simulink model "controlMCUSlugsMKII"  (Simulink 6.6)
settings: Solver=FixedStepDiscrete  StartTime=0.0  StopTime=10.0  FixedStep=0.01  RelTol=1e-3
InitFcn:
  | mcuInit
values from neighbouring files (symbols this model uses):
  apSampleTime = 0.01    [mcuInit.m]
  derivativesConstant = 5    [mcuInit.m]
  T = 0.01    [mcuInit.m]
undefined symbols (not defined in the file or in its folder): bankCommandLimit, baseHeight, bda, bde, bdr, bdt, bICda, bICde, bICdr, bICdt, controlMCUInit, daLimit, deLimit, drLimit, dtLimit, getAccBias, getAccels, getAttitude, getMidLevelCommands, getPassValues, getPidIdx, getVned, getWP, getXYZ, gsRead, ISA_g, lowRateTelemetryMavlink, mda, mde, mdr, mdt, mICda, mICde, mICdr, mICdt, pitchCommandLimit, protDecodeMavlink, readIpc, send2GS, setCurrentCommands, setDiagnosticFloat, setDiagnosticShort, setLogFloat1, setLogFloat2, setNavLat, setNavLong, setNavNav, u1, u2, updateEuler, updateLoad, updatePQR, updatePWM, updatePWM2, y1
libraries: dsPICdrivers x85, simulink x79, SLUGS_Library x23, aerolibconvert2 x5, aerolibutil x3
(part 3 of 5)

== system controlMCUSlugsMKII/Inner Loop/ Navigation/Longitudinal Channel/Protect NaNs ==
  In1 : Inport
  Integer Delay3 : simulink/Discrete/Integer Delay  Orientation=left  vinit=0.0  samptime=T  NumDelays=1
  Relational Operator2 : RelationalOperator  Operator===  LogicOutDataTypeMode=Specify via dialog
  Switch3 : Switch  Criteria=u2 > Threshold  Threshold=0.3  SampleTime=.01
  Out1 : Outport  Orientation=down
  wires:
  Relational Operator2/1 -> Switch3/2
  In1/1 -> Switch3/1, Relational Operator2/1, Relational Operator2/2
  Switch3/1 -> Integer Delay3/1, Out1/1
  Integer Delay3/1 -> Switch3/3

== system controlMCUSlugsMKII/Inner Loop/ Navigation/Longitudinal Channel/Protect NaNs1 ==
  In1 : Inport
  Integer Delay3 : simulink/Discrete/Integer Delay  Orientation=left  vinit=0.0  samptime=T  NumDelays=1
  Relational Operator2 : RelationalOperator  Operator===  LogicOutDataTypeMode=Specify via dialog
  Switch3 : Switch  Criteria=u2 > Threshold  Threshold=0.3  SampleTime=.01
  Out1 : Outport  Orientation=down
  wires:
  Relational Operator2/1 -> Switch3/2
  In1/1 -> Switch3/1, Relational Operator2/1, Relational Operator2/2
  Switch3/1 -> Integer Delay3/1, Out1/1
  Integer Delay3/1 -> Switch3/3

== system controlMCUSlugsMKII/Inner Loop/ Navigation/Longitudinal Channel/Protect NaNs2 ==
  In1 : Inport
  Integer Delay3 : simulink/Discrete/Integer Delay  Orientation=left  vinit=0.0  samptime=T  NumDelays=1
  Relational Operator2 : RelationalOperator  Operator===  LogicOutDataTypeMode=Specify via dialog
  Switch3 : Switch  Criteria=u2 > Threshold  Threshold=0.3  SampleTime=.01
  Out1 : Outport  Orientation=down
  wires:
  Integer Delay3/1 -> Switch3/3
  Switch3/1 -> Out1/1, Integer Delay3/1
  In1/1 -> Relational Operator2/2, Relational Operator2/1, Switch3/1
  Relational Operator2/1 -> Switch3/2

== system controlMCUSlugsMKII/Inner Loop/ Navigation/Longitudinal Channel/Protect NaNs3 ==
  In1 : Inport
  Integer Delay3 : simulink/Discrete/Integer Delay  Orientation=left  vinit=0.0  samptime=T  NumDelays=1
  Relational Operator2 : RelationalOperator  Operator===  LogicOutDataTypeMode=Specify via dialog
  Switch3 : Switch  Criteria=u2 > Threshold  Threshold=0.3  SampleTime=.01
  Out1 : Outport  Orientation=down
  wires:
  Integer Delay3/1 -> Switch3/3
  Switch3/1 -> Out1/1, Integer Delay3/1
  In1/1 -> Relational Operator2/2, Relational Operator2/1, Switch3/1
  Relational Operator2/1 -> Switch3/2

== system controlMCUSlugsMKII/Inner Loop/ Navigation/Longitudinal Channel/Protect NaNs4 ==
  In1 : Inport
  Integer Delay3 : simulink/Discrete/Integer Delay  Orientation=left  vinit=0.0  samptime=T  NumDelays=1
  Relational Operator2 : RelationalOperator  Operator===  LogicOutDataTypeMode=Specify via dialog
  Switch3 : Switch  Criteria=u2 > Threshold  Threshold=0.3  SampleTime=.01
  Out1 : Outport  Orientation=down
  wires:
  Integer Delay3/1 -> Switch3/3
  Switch3/1 -> Out1/1, Integer Delay3/1
  In1/1 -> Relational Operator2/2, Relational Operator2/1, Switch3/1
  Relational Operator2/1 -> Switch3/2

== system controlMCUSlugsMKII/Inner Loop/ Navigation/Longitudinal Channel/Subsystem5 ==
  u : Inport
  C Function Call1 : dsPICdrivers/OTHERS/C Function Call  Tag=dsPIC_dsPIC_CFunctionCall  fctName='myCos'  INPUT_SIZE=1  INPUT1=real32  INPUT2=--  INPUT3=--  OUTPUT_SIZE=1  OUTPUT1=real32  SampleTime=-1  InputType=[ 7 ]  OutputType=[ 7 ]  FctDeclaration=extern real32_T myCos(real32_T u1);  FctCall=%y1 = myCos(%u1);  OrderingInOutPopup=None
  cos(u) : Outport
  wires:
  u/1 -> C Function Call1/1
  C Function Call1/1 -> cos(u)/1

== system controlMCUSlugsMKII/Inner Loop/ Navigation/Navigation/Compute Lateral Error ==
  N : Inport
  WP1 : Inport  Port=2
  UAV pos : Inport  Port=3
  Add : Sum  Inputs=+-  OutScaling=2^-10
  Subsystem3 : Subsystem  AncestorBlock=SLUGS_Library/Subsystem3
  Pe_lat : Outport
  wires:
  Subsystem3/1(x dot y) -> Pe_lat/1
  Add/1 -> Subsystem3/2(y)
  N/1 -> Subsystem3/1(x)
  UAV pos/1 -> Add/2
  WP1/1 -> Add/1

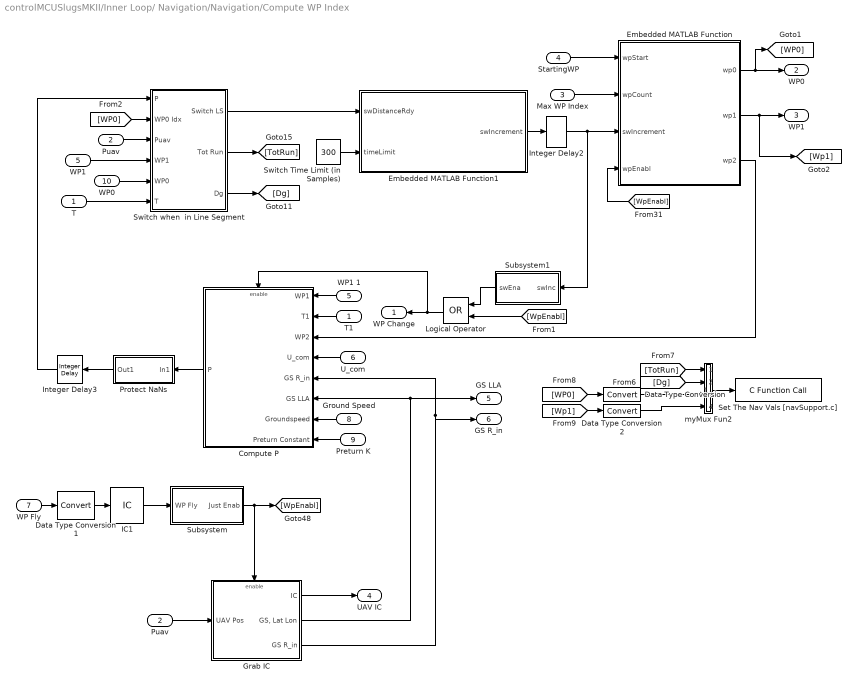
== system controlMCUSlugsMKII/Inner Loop/ Navigation/Navigation/Compute WP Index ==
  T1 : Inport  Orientation=left
  Puav : Inport  Port=2
  Max WP Index : Inport  Port=3
  StartingWP : Inport  Port=4
  "WP1 " : Inport  Port=5
  U_com : Inport  Orientation=left  Port=6
  WP Fly : Inport  Port=7
  Ground Speed : Inport  Orientation=left  Port=8
  Preturn K : Inport  Orientation=left  Port=9
  "WP0 " : Inport  Port=10
  Compute P : Subsystem  Orientation=left
  Data Type Conversion : DataTypeConversion  OutDataTypeMode=single
  Data Type Conversion1 : DataTypeConversion  OutDataTypeMode=double  SampleTime=apSampleTime
  Data Type Conversion2 : DataTypeConversion  OutDataTypeMode=single
  Embedded MATLAB Function : Stateflow chart
  Embedded MATLAB Function1 : Stateflow chart
  Grab IC : Subsystem  TreatAsAtomicUnit=on
  IC1 : InitialCondition  Value=0
  Integer Delay2 : simulink/Discrete/Integer Delay  vinit=1  samptime=-1  NumDelays=1
  Integer Delay3 : simulink/Discrete/Integer Delay  Orientation=left  vinit=50  samptime=-1  NumDelays=1
  Logical Operator : Logic  Orientation=left  Operator=OR  AllPortsSameDT=off  OutDataTypeMode=Boolean
  Protect NaNs : Subsystem  Orientation=left
  "Puav " : InportShadow  Port=2  LatchByCopyingInsideSignal=off
  Set The Nav Vals [navSupport.c] : dsPICdrivers/OTHERS/C Function Call  Tag=dsPIC_dsPIC_CFunctionCall  fctName='setNavNav'  INPUT_SIZE=4  INPUT1=real32  INPUT2=--  INPUT3=--  OUTPUT_SIZE=1  OUTPUT1=--  SampleTime=.01  InputType=[ 7 ]  OutputType=[ ]  FctDeclaration=extern void setNavNav(real32_T* u1);  FctCall=setNavNav(*%u1);  OrderingInOutPopup=None
  Subsystem : Subsystem
  Subsystem1 : Subsystem  Orientation=left
  Switch Time Limit (in Samples) : Constant  Value=300  OutDataTypeMode=single
  Switch when  in Line Segment : Subsystem
  "T " : InportShadow  Port=1  LatchByCopyingInsideSignal=off
  WP1 1 : InportShadow  Orientation=left  Port=5  LatchByCopyingInsideSignal=off
  myMux Fun2 : Stateflow chart
  WP Change : Outport  Orientation=left
  WP0 : Outport  Port=2
  WP1 : Outport  Port=3
  UAV IC : Outport  Port=4
  GS LLA : Outport  Port=5
  GS R_in : Outport  Port=6
  wires:
  Subsystem1/1(swEna) -> Logical Operator/1
  Switch Time Limit (in Samples)/1 -> Embedded MATLAB Function1/2(timeLimit)
  Switch when  in Line Segment/1(Switch LS) -> Embedded MATLAB Function1/1(swDistanceRdy)
  [WpEnabl] -> Logical Operator/2
  Embedded MATLAB Function1/1(swIncrement) -> Integer Delay2/1
  Grab IC/3(GS R_in) -> GS R_in/1, Compute P/5(GS R_in)
  Grab IC/2("GS, Lat Lon") -> GS LLA/1, Compute P/6(GS LLA)
  Logical Operator/1 -> WP Change/1, Compute P/Enable
  [WpEnabl] -> Embedded MATLAB Function/4(wpEnabl)
  IC1/1 -> Subsystem/1(WP Fly)
  Grab IC/1(IC) -> UAV IC/1
  "Puav "/1 -> Grab IC/1(UAV Pos)
  Subsystem/1(Just Enab) -> Grab IC/Enable, [WpEnabl]
  WP Fly/1 -> Data Type Conversion1/1
  U_com/1 -> Compute P/4(U_com)
  Compute P/1(P) -> Protect NaNs/1(In1)
  T1/1 -> Compute P/2(T1)
  WP1 1/1 -> Compute P/1(WP1)
  Embedded MATLAB Function/3(wp2) -> Compute P/3(WP2)
  Max WP Index/1 -> Embedded MATLAB Function/2(wpCount)
  StartingWP/1 -> Embedded MATLAB Function/1(wpStart)
  Embedded MATLAB Function/1(wp0) -> [WP0], WP0/1
  Embedded MATLAB Function/2(wp1) -> WP1/1, [Wp1]
  Data Type Conversion1/1 -> IC1/1
  Ground Speed/1 -> Compute P/7(Groundspeed)
  Preturn K/1 -> Compute P/8(Preturn Constant)
  [WP0] -> Switch when  in Line Segment/2(WP0 Idx)
  Puav/1 -> Switch when  in Line Segment/3(Puav)
  Integer Delay3/1 -> Switch when  in Line Segment/1(P)
  "WP1 "/1 -> Switch when  in Line Segment/4("WP1 ")
  "T "/1 -> Switch when  in Line Segment/6(T)
  "WP0 "/1 -> Switch when  in Line Segment/5(WP0)
  Switch when  in Line Segment/2(Tot Run) -> [TotRun]
  Switch when  in Line Segment/3(Dg) -> [Dg]
  Integer Delay2/1 -> Embedded MATLAB Function/3(swIncrement), Subsystem1/1(swInc)
  myMux Fun2/1(y) -> Set The Nav Vals [navSupport.c]/1
  [TotRun] -> myMux Fun2/1(u1)
  [Dg] -> myMux Fun2/2(u2)
  [WP0] -> Data Type Conversion/1
  Data Type Conversion/1 -> myMux Fun2/3(u3)
  [Wp1] -> Data Type Conversion2/1
  Data Type Conversion2/1 -> myMux Fun2/4(u4)
  Protect NaNs/1(Out1) -> Integer Delay3/1

== system controlMCUSlugsMKII/Inner Loop/ Navigation/Navigation/Get Wps Compute Frenet ==
  WP Idx 0 : Inport
  WP Idx 1 : Inport  Port=2
  UAV IC : Inport  Port=3
  GS LLA : Inport  Port=4
  GS R_in : Inport  Port=5
  Enable : EnablePort
  Compute Frenet : SLUGS_Library/Navigation/Compute Frenet  SystemSampleTime=-1
  Demux : Demux  Outputs=3
  Demux1 : Demux  Outputs=3
  "GS LLA " : InportShadow  Port=4  LatchByCopyingInsideSignal=off
  "GS R_in " : InportShadow  Port=5  LatchByCopyingInsideSignal=off
  Geod2LTP1 : Subsystem
      mask Description:
      | This block provides transformation of the Geodetic coordinates
      | to the LTP coorinate system. The block uses two consecutive transformations
      | (Geodetic -> ECEF ->LTP).
      | Geodetic coordinates of the LTP origin should also be predetermined.
      mask Help: Oops!
      mask Display: plot(0,0,100,100,[45,40,35,40,40],[85,95,85,95,40],[85,95,85,95,40],[35,40,45,40,40],[60,40,10,20,10,14],[70,40,10,13,10,20],[56,45],[70,70],[60,60],[50,60],[60,60],[30,40],[50,60],[20,20],[30,40],[20,20],[45,55],[35,25],[75,65],[35,25])
  Geod2LTP2 : Subsystem
      mask Description:
      | This block provides transformation of the Geodetic coordinates
      | to the LTP coorinate system. The block uses two consecutive transformations
      | (Geodetic -> ECEF ->LTP).
      | Geodetic coordinates of the LTP origin should also be predetermined.
      mask Help: Oops!
      mask Display: plot(0,0,100,100,[45,40,35,40,40],[85,95,85,95,40],[85,95,85,95,40],[35,40,45,40,40],[60,40,10,20,10,14],[70,40,10,13,10,20],[56,45],[70,70],[60,60],[50,60],[60,60],[30,40],[50,60],[20,20],[30,40],[20,20],[45,55],[35,25],[75,65],[35,25])
  Switch : Switch  Criteria=u2 > Threshold  Threshold=0.3
  get WP Coord from Index : Subsystem  AncestorBlock=SLUGS_Library/Navigation/get WP Coord from Index
  "get WP Coord from Index " : Subsystem  AncestorBlock=SLUGS_Library/Navigation/get WP Coord from Index
  T : Outport
  N : Outport  Port=2
  WP 1 : Outport  Port=3
  WP 0 : Outport  Port=4
  wires:
  Geod2LTP1/1("NEU, m") -> WP 1/1, Compute Frenet/2
  "get WP Coord from Index "/1(WP Coord) -> Demux1/1
  "GS R_in "/1 -> Geod2LTP1/2(GS ECEF)
  "GS LLA "/1 -> Geod2LTP1/1(GS Lat,Lon)
  Demux1/3 -> Geod2LTP1/5(Hight,m(GPS))
  Demux1/2 -> Geod2LTP1/4("Lon, deg(GPS)")
  Demux1/1 -> Geod2LTP1/3("Lat, deg(GPS)")
  Geod2LTP2/1("NEU, m") -> Switch/1
  get WP Coord from Index/1(WP Coord) -> Demux/1
  GS R_in/1 -> Geod2LTP2/2(GS ECEF)
  GS LLA/1 -> Geod2LTP2/1(GS Lat,Lon)
  Demux/3 -> Geod2LTP2/5(Hight,m(GPS))
  Demux/2 -> Geod2LTP2/4("Lon, deg(GPS)")
  Demux/1 -> Geod2LTP2/3("Lat, deg(GPS)")
  WP Idx 0/1 -> get WP Coord from Index/1(WP Idx), Switch/2
  Compute Frenet/1 -> T/1
  Compute Frenet/2 -> N/1
  WP Idx 1/1 -> "get WP Coord from Index "/1(WP Idx)
  Switch/1 -> Compute Frenet/1, WP 0/1
  UAV IC/1 -> Switch/3

== system controlMCUSlugsMKII/Inner Loop/ Navigation/Navigation/Park, Deyst & How Lat Accel Cmd ==
  Vxyz : Inport
  T : Inport  Port=2
  N : Inport  Port=3
  Pe_lat : Inport  Port=4
  L2 base : Inport  Port=5
  Lat Accel Gain : Inport  Port=6
  Compute Eta : Subsystem
  Compute L2 Vector LINE MODE : Subsystem
  GainSchedule L2 and Get Groundspeed : Subsystem
  Park's Lateral Accel Command : Subsystem
  Product : Product  RndMeth=Zero
  Set Log Floats 1-3 [navSupport.c] : dsPICdrivers/OTHERS/C Function Call  Tag=dsPIC_dsPIC_CFunctionCall  fctName='setLogFloat1'  INPUT_SIZE=3  INPUT1=real32  INPUT2=--  INPUT3=--  OUTPUT_SIZE=1  OUTPUT1=--  SampleTime=.01  InputType=[ 7 ]  OutputType=[ ]  FctDeclaration=extern void setLogFloat1(real32_T* u1);  FctCall=setLogFloat1(*%u1);  OrderingInOutPopup=None
  "Vxyz " : InportShadow  Port=1  LatchByCopyingInsideSignal=off
  a_s_c : Outport
  Groundspeed : Outport  Orientation=left  Port=2
  wires:
  N/1 -> Compute L2 Vector LINE MODE/4(N)
  T/1 -> Compute L2 Vector LINE MODE/3(T)
  GainSchedule L2 and Get Groundspeed/1(L2) -> Compute L2 Vector LINE MODE/2(L2), Park's Lateral Accel Command/1(L2)
  Pe_lat/1 -> Compute L2 Vector LINE MODE/1(Pe_lat)
  Vxyz/1 -> Compute Eta/1(Vxyz)
  Compute Eta/1(Eta) -> Park's Lateral Accel Command/2(eta)
  Compute L2 Vector LINE MODE/1(L2_vec) -> Compute Eta/2(L2_vec), Set Log Floats 1-3 [navSupport.c]/1
  Park's Lateral Accel Command/1(a_s_c) -> Product/2
  L2 base/1 -> GainSchedule L2 and Get Groundspeed/1(L2 Base)
  GainSchedule L2 and Get Groundspeed/2(Ground Speed) -> Groundspeed/1, Compute Eta/3(Ground Speed), Park's Lateral Accel Command/3(Ground Speed)
  "Vxyz "/1 -> GainSchedule L2 and Get Groundspeed/2(Vxyz)
  Lat Accel Gain/1 -> Product/1
  Product/1 -> a_s_c/1

== system controlMCUSlugsMKII/Inner Loop/ Navigation/Navigation/as_c to phi_c ==
  as_c : Inport
  g : Inport  Port=2
  Divide : Product  Inputs=*/  OutScaling=2^-10
  Protect NaNs : Subsystem
  Subsystem2 : SLUGS_Library/Subsystem2  SystemSampleTime=-1
  phi_c : Outport
  wires:
  g/1 -> Divide/2
  Subsystem2/1 -> Protect NaNs/1(In1)
  as_c/1 -> Divide/1
  Divide/1 -> Subsystem2/1
  Protect NaNs/1(Out1) -> phi_c/1

== system controlMCUSlugsMKII/Trim Vals/Grab I.C./Convert to Rad ==
  IC : Inport  Orientation=down
  Add : Sum  OutScaling=2^-10
  Constant1 : Constant  Value=slopem
  Constant2 : Constant  Value=interceptb
  Data Type Conversion : DataTypeConversion  OutDataTypeMode=single
  Divide : Product  OutScaling=2^-10
  Angle (rad) : Outport
  wires:
  Data Type Conversion/1 -> Angle (rad)/1
  IC/1 -> Divide/1
  Constant2/1 -> Add/2
  Divide/1 -> Add/1
  Add/1 -> Data Type Conversion/1
  Constant1/1 -> Divide/2

== system controlMCUSlugsMKII/Trim Vals/Grab I.C./Convert to Rad1 ==
  IC : Inport  Orientation=down
  Add : Sum  OutScaling=2^-10
  Constant1 : Constant  Value=slopem
  Constant2 : Constant  Value=interceptb
  Data Type Conversion : DataTypeConversion  OutDataTypeMode=single
  Divide : Product  OutScaling=2^-10
  Angle (rad) : Outport
  wires:
  Constant1/1 -> Divide/2
  Add/1 -> Data Type Conversion/1
  Divide/1 -> Add/1
  Constant2/1 -> Add/2
  IC/1 -> Divide/1
  Data Type Conversion/1 -> Angle (rad)/1

== system controlMCUSlugsMKII/Trim Vals/Grab I.C./Convert to Rad2 ==
  IC : Inport  Orientation=down
  Add : Sum  OutScaling=2^-10
  Constant1 : Constant  Value=slopem
  Constant2 : Constant  Value=interceptb
  Data Type Conversion : DataTypeConversion  OutDataTypeMode=single
  Divide : Product  OutScaling=2^-10
  Angle (rad) : Outport
  wires:
  Data Type Conversion/1 -> Angle (rad)/1
  IC/1 -> Divide/1
  Constant2/1 -> Add/2
  Divide/1 -> Add/1
  Add/1 -> Data Type Conversion/1
  Constant1/1 -> Divide/2

== system controlMCUSlugsMKII/Trim Vals/Grab I.C./Convert to Rad3 ==
  IC : Inport  Orientation=down
  Add : Sum  OutScaling=2^-10
  Constant1 : Constant  Value=slopem
  Constant2 : Constant  Value=interceptb
  Data Type Conversion : DataTypeConversion  OutDataTypeMode=single
  Divide : Product  OutScaling=2^-10
  Angle (rad) : Outport
  wires:
  Constant1/1 -> Divide/2
  Add/1 -> Data Type Conversion/1
  Divide/1 -> Add/1
  Constant2/1 -> Add/2
  IC/1 -> Divide/1
  Data Type Conversion/1 -> Angle (rad)/1

== system controlMCUSlugsMKII/Trim Vals/Log  Trims Using PWM High [groundStationDriver.c]/Report Airspeed ==
  Um : Inport  Orientation=down
  Data Type Conversion4 : DataTypeConversion  OutDataTypeMode=uint16  SampleTime=apSampleTime  SaturateOnIntegerOverflow=on
  Gain4 : Gain  Gain=1000
  Update PWM  Commands4 : dsPICdrivers/OTHERS/C Function Call  Tag=dsPIC_dsPIC_CFunctionCall  fctName='updatePWM2'  INPUT_SIZE=1  INPUT1=uint16  INPUT2=uint8  INPUT3=--  OUTPUT_SIZE=1  OUTPUT1=--  SampleTime=-1  InputType=[ 4 2 ]  OutputType=[ ]  FctDeclaration=extern void updatePWM2(uint16_T u1, uint8_T u2);  FctCall=updatePWM2(%u1, %u2);  OrderingInOutPopup=None
  dlf1 : Constant  Value=4  OutDataTypeMode=uint8
  wires:
  Data Type Conversion4/1 -> Update PWM  Commands4/1
  dlf1/1 -> Update PWM  Commands4/2
  Gain4/1 -> Data Type Conversion4/1
  Um/1 -> Gain4/1

== system controlMCUSlugsMKII/Update PWM Commands and Send Telemetry/Generate PWM Signals Based on the Control Type/If  Control Type Is Manual ==
  Pilot (IC) : Inport
  Action Port : ActionPort  ActionType=then
  Demux : Demux
  Gain{,1..3} (4 alike) : Gain  Gain=0.5
  myMux Fun1 : Stateflow chart
  PWM : Outport
  wires:
  Gain/1 -> myMux Fun1/1(u1)
  Gain1/1 -> myMux Fun1/2(u2)
  Gain2/1 -> myMux Fun1/3(u3)
  Gain3/1 -> myMux Fun1/4(u4)
  Demux/1 -> Gain/1
  Demux/2 -> Gain1/1
  Demux/3 -> Gain2/1
  Demux/4 -> Gain3/1
  myMux Fun1/1(y) -> PWM/1
  Pilot (IC)/1 -> Demux/1

== system controlMCUSlugsMKII/Update PWM Commands and Send Telemetry/Generate PWM Signals Based on the Control Type/If  Control Type Is Passthrough ==
  Pilot (IC) : Inport
  Action Port : ActionPort  ActionType=elseif
  Demux : Demux
  Gain{,1..3} (4 alike) : Gain  Gain=0.5
  myMux Fun1 : Stateflow chart
  PWM (abs) : Outport
  wires:
  Gain/1 -> myMux Fun1/1(u1)
  Gain1/1 -> myMux Fun1/2(u2)
  Gain2/1 -> myMux Fun1/3(u3)
  Gain3/1 -> myMux Fun1/4(u4)
  Demux/1 -> Gain/1
  Demux/2 -> Gain1/1
  Demux/3 -> Gain2/1
  Demux/4 -> Gain3/1
  myMux Fun1/1(y) -> PWM (abs)/1
  Pilot (IC)/1 -> Demux/1

== system controlMCUSlugsMKII/Update PWM Commands and Send Telemetry/Generate PWM Signals Based on the Control Type/If  Control Type Is Selective Passthrough ==
  PWM(rad) : Inport
  Pilot (IC) : Inport  Port=2
  Action Port : ActionPort  ActionType=elseif
  Convert to PWM : Subsystem  mask{slopem=mde, interceptb=bde}
      mask prompts: slopem "Slope"; interceptb "Intercept"
  Convert to PWM1 : Subsystem  mask{slopem=mdt, interceptb=bdt}
      mask prompts: slopem "Slope"; interceptb "Intercept"
  Convert to PWM2 : Subsystem  mask{slopem=mda, interceptb=bda}
      mask prompts: slopem "Slope"; interceptb "Intercept"
  Convert to PWM3 : Subsystem  mask{slopem=mdr, interceptb=bdr}
      mask prompts: slopem "Slope"; interceptb "Intercept"
  Demux : Demux  Orientation=down
  Demux1 : Demux
  Demux2 : Demux
  Gain{,1..3} (4 alike) : Gain  Gain=0.5
  Get Pass Switches [navSupport.c] : dsPICdrivers/OTHERS/C Function Call  Tag=dsPIC_dsPIC_CFunctionCall  fctName='getPassValues'  INPUT_SIZE=1  INPUT1=--  INPUT2=--  INPUT3=--  OUTPUT_SIZE=4  OUTPUT1=uint8  SampleTime=.01  InputType=[ ]  OutputType=[ 2 ]  FctDeclaration=extern void getPassValues(uint8_T* y1);  FctCall=getPassValues(*%y1);  OrderingInOutPopup=None
  Switch{,1..3} (4 alike) : Switch  Threshold=0.5
  myMux Fun1 : Stateflow chart
  PWM : Outport
  wires:
  myMux Fun1/1(y) -> PWM/1
  Switch/1 -> myMux Fun1/1(u1)
  Switch1/1 -> myMux Fun1/2(u2)
  Switch2/1 -> myMux Fun1/3(u3)
  Switch3/1 -> myMux Fun1/4(u4)
  Get Pass Switches [navSupport.c]/1 -> Demux/1
  Demux/4 -> Switch/2
  Demux/3 -> Switch1/2
  Demux/2 -> Switch2/2
  Demux/1 -> Switch3/2
  Demux1/1 -> Convert to PWM1/1(" Angle(rad)")
  Demux1/2 -> Convert to PWM2/1(" Angle(rad)")
  Demux1/3 -> Convert to PWM3/1(" Angle(rad)")
  Demux1/4 -> Convert to PWM/1(" Angle(rad)")
  PWM(rad)/1 -> Demux1/1
  Convert to PWM1/1(PWM) -> Switch/3
  Convert to PWM2/1(PWM) -> Switch1/3
  Convert to PWM3/1(PWM) -> Switch2/3
  Convert to PWM/1(PWM) -> Switch3/3
  Demux2/1 -> Gain/1
  Demux2/2 -> Gain1/1
  Demux2/3 -> Gain2/1
  Demux2/4 -> Gain3/1
  Pilot (IC)/1 -> Demux2/1
  Gain/1 -> Switch/1
  Gain1/1 -> Switch1/1
  Gain2/1 -> Switch2/1
  Gain3/1 -> Switch3/1

== system controlMCUSlugsMKII/Update PWM Commands and Send Telemetry/Generate PWM Signals Based on the Control Type/If  Control Type Is Wp Follow  or Inner Cmds ==
  PWM(rad) : Inport
  Action Port : ActionPort  ActionType=elseif
  Convert to PWM : Subsystem  mask{slopem=mde, interceptb=bde}
      mask prompts: slopem "Slope"; interceptb "Intercept"
  Convert to PWM1 : Subsystem  mask{slopem=mdt, interceptb=bdt}
      mask prompts: slopem "Slope"; interceptb "Intercept"
  Convert to PWM2 : Subsystem  mask{slopem=mda, interceptb=bda}
      mask prompts: slopem "Slope"; interceptb "Intercept"
  Convert to PWM3 : Subsystem  mask{slopem=mdr, interceptb=bdr}
      mask prompts: slopem "Slope"; interceptb "Intercept"
  Demux : Demux
  myMux Fun1 : Stateflow chart
  PWM (abs) : Outport
  wires:
  myMux Fun1/1(y) -> PWM (abs)/1
  Convert to PWM1/1(PWM) -> myMux Fun1/1(u1)
  Convert to PWM2/1(PWM) -> myMux Fun1/2(u2)
  Convert to PWM3/1(PWM) -> myMux Fun1/3(u3)
  Convert to PWM/1(PWM) -> myMux Fun1/4(u4)
  Demux/1 -> Convert to PWM1/1(" Angle(rad)")
  Demux/2 -> Convert to PWM2/1(" Angle(rad)")
  Demux/3 -> Convert to PWM3/1(" Angle(rad)")
  Demux/4 -> Convert to PWM/1(" Angle(rad)")
  PWM(rad)/1 -> Demux/1

== system controlMCUSlugsMKII/get Nav Vars/Direction Cosine Matrix to Euler Angles/Subsystem1 ==
  u : Inport
  v : Inport  Port=2
  C Function Call : dsPICdrivers/OTHERS/C Function Call  Tag=dsPIC_dsPIC_CFunctionCall  fctName='myAtan2'  INPUT_SIZE=1  INPUT1=real32  INPUT2=real32  INPUT3=--  OUTPUT_SIZE=1  OUTPUT1=real32  SampleTime=-1  InputType=[ 7 7 ]  OutputType=[ 7 ]  FctDeclaration=extern real32_T myAtan2(real32_T u1, real32_T u2);  FctCall=%y1 = myAtan2(%u1, %u2);  OrderingInOutPopup=None
  atan2(x,y) : Outport
  wires:
  C Function Call/1 -> atan2(x,y)/1
  v/1 -> C Function Call/2
  u/1 -> C Function Call/1

== system controlMCUSlugsMKII/get Nav Vars/Direction Cosine Matrix to Euler Angles/Subsystem2 ==
  u : Inport
  v : Inport  Port=2
  C Function Call : dsPICdrivers/OTHERS/C Function Call  Tag=dsPIC_dsPIC_CFunctionCall  fctName='myAtan2'  INPUT_SIZE=1  INPUT1=real32  INPUT2=real32  INPUT3=--  OUTPUT_SIZE=1  OUTPUT1=real32  SampleTime=-1  InputType=[ 7 7 ]  OutputType=[ 7 ]  FctDeclaration=extern real32_T myAtan2(real32_T u1, real32_T u2);  FctCall=%y1 = myAtan2(%u1, %u2);  OrderingInOutPopup=None
  atan2(x,y) : Outport
  wires:
  u/1 -> C Function Call/1
  v/1 -> C Function Call/2
  C Function Call/1 -> atan2(x,y)/1

== system controlMCUSlugsMKII/get Nav Vars/Direction Cosine Matrix to Euler Angles/Subsystem3 ==
  x : Inport
  C Function Call : dsPICdrivers/OTHERS/C Function Call  Tag=dsPIC_dsPIC_CFunctionCall  fctName='myAsin'  INPUT_SIZE=1  INPUT1=real32  INPUT2=--  INPUT3=--  OUTPUT_SIZE=1  OUTPUT1=real32  SampleTime=-1  InputType=[ 7 ]  OutputType=[ 7 ]  FctDeclaration=extern real32_T myAsin(real32_T u1);  FctCall=%y1 = myAsin(%u1);  OrderingInOutPopup=None
  "[-1,1]" : Saturate  UpperLimit=0.9999  LowerLimit=-0.999
  asin(x) : Outport
  wires:
  C Function Call/1 -> asin(x)/1
  x/1 -> "[-1,1]"/1
  "[-1,1]"/1 -> C Function Call/1

== system controlMCUSlugsMKII/get Nav Vars/Direction Cosine Matrix to Euler Angles/cos(phi)cos(theta) ==
  DCM : Inport
  Demux : Demux  Outputs=9
  Terminator{,1..7} (8 alike) : Terminator
  cos(phi)cos(theta) : Outport
  wires:
  Demux/4 -> Terminator/1
  Demux/3 -> Terminator1/1
  Demux/5 -> Terminator4/1
  Demux/2 -> Terminator3/1
  Demux/1 -> Terminator2/1
  DCM/1 -> Demux/1
  Demux/8 -> Terminator7/1
  Demux/6 -> Terminator5/1
  Demux/7 -> Terminator6/1
  Demux/9 -> cos(phi)cos(theta)/1

== system controlMCUSlugsMKII/get Nav Vars/Direction Cosine Matrix to Euler Angles/cos(psi)cos(theta) ==
  DCM : Inport
  Demux : Demux  Outputs=9
  Terminator{,1..7} (8 alike) : Terminator
  cos(psi)cos(theta) : Outport
  wires:
  Demux/9 -> Terminator2/1
  Demux/7 -> Terminator6/1
  Demux/6 -> Terminator5/1
  Demux/8 -> Terminator7/1
  DCM/1 -> Demux/1
  Demux/1 -> cos(psi)cos(theta)/1
  Demux/2 -> Terminator3/1
  Demux/5 -> Terminator4/1
  Demux/3 -> Terminator1/1
  Demux/4 -> Terminator/1

== system controlMCUSlugsMKII/get Nav Vars/Direction Cosine Matrix to Euler Angles/sin(phi)cos(theta) ==
  DCM : Inport
  Demux : Demux  Outputs=9
  Terminator{,1..7} (8 alike) : Terminator
  sin(phi)cos(theta) : Outport
  wires:
  Demux/9 -> Terminator7/1
  Demux/7 -> Terminator6/1
  Demux/6 -> Terminator5/1
  Demux/8 -> sin(phi)cos(theta)/1
  DCM/1 -> Demux/1
  Demux/1 -> Terminator2/1
  Demux/2 -> Terminator3/1
  Demux/5 -> Terminator4/1
  Demux/3 -> Terminator1/1
  Demux/4 -> Terminator/1

== system controlMCUSlugsMKII/get Nav Vars/Direction Cosine Matrix to Euler Angles/sin(psi)cos(theta) ==
  DCM : Inport
  Demux : Demux  Outputs=9
  Terminator{,1..7} (8 alike) : Terminator
  sin(psi)cos(theta) : Outport
  wires:
  Demux/4 -> sin(psi)cos(theta)/1
  Demux/3 -> Terminator1/1
  Demux/5 -> Terminator4/1
  Demux/2 -> Terminator3/1
  Demux/1 -> Terminator2/1
  DCM/1 -> Demux/1
  Demux/8 -> Terminator/1
  Demux/6 -> Terminator5/1
  Demux/7 -> Terminator6/1
  Demux/9 -> Terminator7/1

== system controlMCUSlugsMKII/get Nav Vars/Direction Cosine Matrix to Euler Angles/sin(theta) ==
  DCM : Inport
  Demux : Demux  Outputs=9
  Gain2 : Gain  Gain=-1  SaturateOnIntegerOverflow=on
  Terminator{,1..5,7..8} (8 alike) : Terminator
  sin(theta) : Outport
  wires:
  Gain2/1 -> sin(theta)/1
  Demux/4 -> Terminator/1
  Demux/3 -> Terminator1/1
  Demux/5 -> Terminator4/1
  Demux/2 -> Terminator3/1
  Demux/1 -> Terminator2/1
  DCM/1 -> Demux/1
  Demux/8 -> Terminator8/1
  Demux/6 -> Terminator5/1
  Demux/7 -> Gain2/1
  Demux/9 -> Terminator7/1

== system controlMCUSlugsMKII/get Nav Vars/Euler Angles to  Direction Cosine Matrix1/A11 ==
  sin_cos : Inport
  Demux : Demux  Outputs=6
  Terminator{,1..3} (4 alike) : Terminator
  u(5)*u(6) : Product  RndMeth=Zero
  A11 : Outport
  wires:
  Demux/6 -> u(5)*u(6)/2
  u(5)*u(6)/1 -> A11/1
  sin_cos/1 -> Demux/1
  Demux/1 -> Terminator2/1
  Demux/2 -> Terminator3/1
  Demux/5 -> u(5)*u(6)/1
  Demux/3 -> Terminator1/1
  Demux/4 -> Terminator/1

== system controlMCUSlugsMKII/get Nav Vars/Euler Angles to  Direction Cosine Matrix1/A12 ==
  sin_cos : Inport
  Demux : Demux  Outputs=6
  Terminator{,1..3} (4 alike) : Terminator
  u(3)*u(5) : Product  RndMeth=Zero
  A12 : Outport
  wires:
  Demux/4 -> Terminator/1
  Demux/3 -> u(3)*u(5)/1
  Demux/5 -> u(3)*u(5)/2
  Demux/2 -> Terminator3/1
  Demux/1 -> Terminator2/1
  sin_cos/1 -> Demux/1
  u(3)*u(5)/1 -> A12/1
  Demux/6 -> Terminator1/1

== system controlMCUSlugsMKII/get Nav Vars/Euler Angles to  Direction Cosine Matrix1/A13 ==
  sin_cos : Inport
  Demux : Demux  Outputs=6
  Gain2 : Gain  Gain=-1  SaturateOnIntegerOverflow=on
  Terminator{,1..4} (5 alike) : Terminator
  A13 : Outport
  wires:
  Demux/6 -> Terminator1/1
  sin_cos/1 -> Demux/1
  Demux/1 -> Terminator2/1
  Demux/2 -> Gain2/1
  Demux/5 -> Terminator4/1
  Demux/3 -> Terminator3/1
  Demux/4 -> Terminator/1
  Gain2/1 -> A13/1

== system controlMCUSlugsMKII/get Nav Vars/Euler Angles to  Direction Cosine Matrix1/A21 ==
  sin_cos : Inport
  Demux : Demux  Outputs=6
  Sum : Sum  Inputs=|+-
  Terminator : Terminator
  u(3)*u(4) : Product  RndMeth=Zero
  u(6)*u(1)*u(2) : Product  Inputs=3  RndMeth=Zero
  A21 : Outport
  wires:
  Sum/1 -> A21/1
  u(3)*u(4)/1 -> Sum/2
  u(6)*u(1)*u(2)/1 -> Sum/1
  sin_cos/1 -> Demux/1
  Demux/1 -> u(6)*u(1)*u(2)/2
  Demux/2 -> u(6)*u(1)*u(2)/3
  Demux/5 -> Terminator/1
  Demux/6 -> u(6)*u(1)*u(2)/1
  Demux/3 -> u(3)*u(4)/1
  Demux/4 -> u(3)*u(4)/2

== system controlMCUSlugsMKII/get Nav Vars/Euler Angles to  Direction Cosine Matrix1/A22 ==
  sin_cos : Inport
  Demux : Demux  Outputs=6
  Sum : Sum  Inputs=|++
  Terminator : Terminator
  u(1)*u(2)*u(3) : Product  Inputs=3  RndMeth=Zero
  u(4)*u(6) : Product  RndMeth=Zero
  A22 : Outport
  wires:
  Demux/4 -> u(4)*u(6)/1
  Demux/3 -> u(1)*u(2)*u(3)/3
  Demux/5 -> Terminator/1
  Demux/2 -> u(1)*u(2)*u(3)/2
  Demux/1 -> u(1)*u(2)*u(3)/1
  sin_cos/1 -> Demux/1
  u(1)*u(2)*u(3)/1 -> Sum/1
  u(4)*u(6)/1 -> Sum/2
  Sum/1 -> A22/1
  Demux/6 -> u(4)*u(6)/2

== system controlMCUSlugsMKII/get Nav Vars/Euler Angles to  Direction Cosine Matrix1/A23 ==
  sin_cos : Inport
  Demux : Demux  Outputs=6
  Terminator{,1..3} (4 alike) : Terminator
  u(1)*u(3) : Product  RndMeth=Zero
  A23 : Outport
  wires:
  Demux/6 -> Terminator1/1
  u(1)*u(3)/1 -> A23/1
  sin_cos/1 -> Demux/1
  Demux/1 -> u(1)*u(3)/1
  Demux/2 -> Terminator3/1
  Demux/5 -> u(1)*u(3)/2
  Demux/3 -> Terminator2/1
  Demux/4 -> Terminator/1

== system controlMCUSlugsMKII/get Nav Vars/Euler Angles to  Direction Cosine Matrix1/A31 ==
  sin_cos : Inport
  Demux : Demux  Outputs=6
  Sum : Sum  Inputs=|++
  Terminator : Terminator
  u(1)*u(3) : Product  RndMeth=Zero
  u(2)*u(4)*u(6) : Product  Inputs=3  RndMeth=Zero
  A31 : Outport
  wires:
  Demux/4 -> u(2)*u(4)*u(6)/2
  Demux/3 -> u(1)*u(3)/2
  Demux/5 -> Terminator/1
  Demux/2 -> u(2)*u(4)*u(6)/1
  Demux/1 -> u(1)*u(3)/1
  sin_cos/1 -> Demux/1
  u(2)*u(4)*u(6)/1 -> Sum/2
  Sum/1 -> A31/1
  Demux/6 -> u(2)*u(4)*u(6)/3
  u(1)*u(3)/1 -> Sum/1

== system controlMCUSlugsMKII/get Nav Vars/Euler Angles to  Direction Cosine Matrix1/A32 ==
  sin_cos : Inport
  Demux : Demux  Outputs=6
  Sum : Sum  Inputs=|+-
  Terminator : Terminator
  u(1)*u(6) : Product  RndMeth=Zero
  u(2)*u(3)*u(4) : Product  Inputs=3  RndMeth=Zero
  A32 : Outport
  wires:
  Demux/6 -> u(1)*u(6)/1
  Sum/1 -> A32/1
  u(1)*u(6)/1 -> Sum/2
  u(2)*u(3)*u(4)/1 -> Sum/1
  sin_cos/1 -> Demux/1
  Demux/1 -> u(1)*u(6)/2
  Demux/2 -> u(2)*u(3)*u(4)/1
  Demux/5 -> Terminator/1
  Demux/3 -> u(2)*u(3)*u(4)/2
  Demux/4 -> u(2)*u(3)*u(4)/3

== system controlMCUSlugsMKII/get Nav Vars/Euler Angles to  Direction Cosine Matrix1/A33 ==
  sin_cos : Inport
  Demux : Demux  Outputs=6
  Terminator{,1..3} (4 alike) : Terminator
  u(4)*u(5) : Product  RndMeth=Zero
  A33 : Outport
  wires:
  Demux/4 -> u(4)*u(5)/1
  Demux/3 -> Terminator1/1
  Demux/5 -> u(4)*u(5)/2
  Demux/2 -> Terminator3/1
  Demux/1 -> Terminator2/1
  sin_cos/1 -> Demux/1
  u(4)*u(5)/1 -> A33/1
  Demux/6 -> Terminator/1

== system controlMCUSlugsMKII/get Nav Vars/Euler Angles to  Direction Cosine Matrix1/Create Transformation Matrix ==
  M11 : Inport
  M12 : Inport  Port=2
  M13 : Inport  Port=3
  M21 : Inport  Port=4
  M22 : Inport  Port=5
  M23 : Inport  Port=6
  M31 : Inport  Port=7
  M32 : Inport  Port=8
  M33 : Inport  Port=9
  Reshape (9) to [3x3] column-major : Reshape  OutputDimensionality=Customize  OutputDimensions=[3,3]
  myMux Fun1 : Stateflow chart
  Matrix : Outport
  wires:
  myMux Fun1/1(y) -> Reshape (9) to [3x3] column-major/1
  M11/1 -> myMux Fun1/1(u1)
  M21/1 -> myMux Fun1/2(u2)
  M31/1 -> myMux Fun1/3(u3)
  M12/1 -> myMux Fun1/4(u4)
  M22/1 -> myMux Fun1/5(u5)
  Reshape (9) to [3x3] column-major/1 -> Matrix/1
  M32/1 -> myMux Fun1/6(u6)
  M13/1 -> myMux Fun1/7(u7)
  M23/1 -> myMux Fun1/8(u8)
  M33/1 -> myMux Fun1/9(u9)

== system controlMCUSlugsMKII/get Nav Vars/Euler Angles to  Direction Cosine Matrix1/Subsystem5 ==
  u : Inport
  C Function Call : dsPICdrivers/OTHERS/C Function Call  Tag=dsPIC_dsPIC_CFunctionCall  fctName='mySin'  INPUT_SIZE=1  INPUT1=real32  INPUT2=--  INPUT3=--  OUTPUT_SIZE=1  OUTPUT1=real32  SampleTime=-1  InputType=[ 7 ]  OutputType=[ 7 ]  FctDeclaration=extern real32_T mySin(real32_T u1);  FctCall=%y1 = mySin(%u1);  OrderingInOutPopup=None
  C Function Call1 : dsPICdrivers/OTHERS/C Function Call  Tag=dsPIC_dsPIC_CFunctionCall  fctName='myCos'  INPUT_SIZE=1  INPUT1=real32  INPUT2=--  INPUT3=--  OUTPUT_SIZE=1  OUTPUT1=real32  SampleTime=-1  InputType=[ 7 ]  OutputType=[ 7 ]  FctDeclaration=extern real32_T myCos(real32_T u1);  FctCall=%y1 = myCos(%u1);  OrderingInOutPopup=None
  C Function Call2 : dsPICdrivers/OTHERS/C Function Call  Tag=dsPIC_dsPIC_CFunctionCall  fctName='mySin'  INPUT_SIZE=1  INPUT1=real32  INPUT2=--  INPUT3=--  OUTPUT_SIZE=1  OUTPUT1=real32  SampleTime=-1  InputType=[ 7 ]  OutputType=[ 7 ]  FctDeclaration=extern real32_T mySin(real32_T u1);  FctCall=%y1 = mySin(%u1);  OrderingInOutPopup=None
  C Function Call3 : dsPICdrivers/OTHERS/C Function Call  Tag=dsPIC_dsPIC_CFunctionCall  fctName='mySin'  INPUT_SIZE=1  INPUT1=real32  INPUT2=--  INPUT3=--  OUTPUT_SIZE=1  OUTPUT1=real32  SampleTime=-1  InputType=[ 7 ]  OutputType=[ 7 ]  FctDeclaration=extern real32_T mySin(real32_T u1);  FctCall=%y1 = mySin(%u1);  OrderingInOutPopup=None
  C Function Call4 : dsPICdrivers/OTHERS/C Function Call  Tag=dsPIC_dsPIC_CFunctionCall  fctName='myCos'  INPUT_SIZE=1  INPUT1=real32  INPUT2=--  INPUT3=--  OUTPUT_SIZE=1  OUTPUT1=real32  SampleTime=-1  InputType=[ 7 ]  OutputType=[ 7 ]  FctDeclaration=extern real32_T myCos(real32_T u1);  FctCall=%y1 = myCos(%u1);  OrderingInOutPopup=None
  C Function Call5 : dsPICdrivers/OTHERS/C Function Call  Tag=dsPIC_dsPIC_CFunctionCall  fctName='myCos'  INPUT_SIZE=1  INPUT1=real32  INPUT2=--  INPUT3=--  OUTPUT_SIZE=1  OUTPUT1=real32  SampleTime=-1  InputType=[ 7 ]  OutputType=[ 7 ]  FctDeclaration=extern real32_T myCos(real32_T u1);  FctCall=%y1 = myCos(%u1);  OrderingInOutPopup=None
  Demux : Demux  Outputs=3
  Demux1 : Demux  Outputs=3
  Environment Controller : simulink/Signal Routing/Environment Controller  SystemSampleTime=-1
  Environment Controller1 : simulink/Signal Routing/Environment Controller  SystemSampleTime=-1
  SinCos1 : aerolibutil/SinCos  SystemSampleTime=-1
  myMux Fun1 : Stateflow chart
  myMux Fun2 : Stateflow chart
  sin(u) : Outport
  cos(u) : Outport  Port=2
  wires:
  Environment Controller/1 -> sin(u)/1
  SinCos1/1 -> Environment Controller/1
  u/1 -> SinCos1/1, Demux/1, Demux1/1
  Environment Controller1/1 -> cos(u)/1
  SinCos1/2 -> Environment Controller1/1
  C Function Call/1 -> myMux Fun1/1(u1)
  C Function Call2/1 -> myMux Fun1/2(u2)
  C Function Call3/1 -> myMux Fun1/3(u3)
  C Function Call1/1 -> myMux Fun2/1(u1)
  C Function Call4/1 -> myMux Fun2/2(u2)
  C Function Call5/1 -> myMux Fun2/3(u3)
  Demux/1 -> C Function Call/1
  Demux/2 -> C Function Call2/1
  Demux/3 -> C Function Call3/1
  Demux1/1 -> C Function Call1/1
  Demux1/2 -> C Function Call4/1
  Demux1/3 -> C Function Call5/1
  myMux Fun1/1(y) -> Environment Controller/2
  myMux Fun2/1(y) -> Environment Controller1/2

== system controlMCUSlugsMKII/get Nav Vars/Euler Angles to  Direction Cosine Matrix2/A11 ==
  sin_cos : Inport
  Demux : Demux  Outputs=6
  Terminator{,1..3} (4 alike) : Terminator
  u(5)*u(6) : Product  RndMeth=Zero
  A11 : Outport
  wires:
  Demux/4 -> Terminator/1
  Demux/3 -> Terminator1/1
  Demux/5 -> u(5)*u(6)/1
  Demux/2 -> Terminator3/1
  Demux/1 -> Terminator2/1
  sin_cos/1 -> Demux/1
  u(5)*u(6)/1 -> A11/1
  Demux/6 -> u(5)*u(6)/2

== system controlMCUSlugsMKII/get Nav Vars/Euler Angles to  Direction Cosine Matrix2/A12 ==
  sin_cos : Inport
  Demux : Demux  Outputs=6
  Terminator{,1..3} (4 alike) : Terminator
  u(3)*u(5) : Product  RndMeth=Zero
  A12 : Outport
  wires:
  Demux/6 -> Terminator1/1
  u(3)*u(5)/1 -> A12/1
  sin_cos/1 -> Demux/1
  Demux/1 -> Terminator2/1
  Demux/2 -> Terminator3/1
  Demux/5 -> u(3)*u(5)/2
  Demux/3 -> u(3)*u(5)/1
  Demux/4 -> Terminator/1

== system controlMCUSlugsMKII/get Nav Vars/Euler Angles to  Direction Cosine Matrix2/A13 ==
  sin_cos : Inport
  Demux : Demux  Outputs=6
  Gain2 : Gain  Gain=-1  SaturateOnIntegerOverflow=on
  Terminator{,1..4} (5 alike) : Terminator
  A13 : Outport
  wires:
  Gain2/1 -> A13/1
  Demux/4 -> Terminator/1
  Demux/3 -> Terminator3/1
  Demux/5 -> Terminator4/1
  Demux/2 -> Gain2/1
  Demux/1 -> Terminator2/1
  sin_cos/1 -> Demux/1
  Demux/6 -> Terminator1/1

== system controlMCUSlugsMKII/get Nav Vars/Euler Angles to  Direction Cosine Matrix2/A21 ==
  sin_cos : Inport
  Demux : Demux  Outputs=6
  Sum : Sum  Inputs=|+-
  Terminator : Terminator
  u(3)*u(4) : Product  RndMeth=Zero
  u(6)*u(1)*u(2) : Product  Inputs=3  RndMeth=Zero
  A21 : Outport
  wires:
  Demux/4 -> u(3)*u(4)/2
  Demux/3 -> u(3)*u(4)/1
  Demux/6 -> u(6)*u(1)*u(2)/1
  Demux/5 -> Terminator/1
  Demux/2 -> u(6)*u(1)*u(2)/3
  Demux/1 -> u(6)*u(1)*u(2)/2
  sin_cos/1 -> Demux/1
  u(6)*u(1)*u(2)/1 -> Sum/1
  u(3)*u(4)/1 -> Sum/2
  Sum/1 -> A21/1

== system controlMCUSlugsMKII/get Nav Vars/Euler Angles to  Direction Cosine Matrix2/A22 ==
  sin_cos : Inport
  Demux : Demux  Outputs=6
  Sum : Sum  Inputs=|++
  Terminator : Terminator
  u(1)*u(2)*u(3) : Product  Inputs=3  RndMeth=Zero
  u(4)*u(6) : Product  RndMeth=Zero
  A22 : Outport
  wires:
  Demux/6 -> u(4)*u(6)/2
  Sum/1 -> A22/1
  u(4)*u(6)/1 -> Sum/2
  u(1)*u(2)*u(3)/1 -> Sum/1
  sin_cos/1 -> Demux/1
  Demux/1 -> u(1)*u(2)*u(3)/1
  Demux/2 -> u(1)*u(2)*u(3)/2
  Demux/5 -> Terminator/1
  Demux/3 -> u(1)*u(2)*u(3)/3
  Demux/4 -> u(4)*u(6)/1

== system controlMCUSlugsMKII/get Nav Vars/Euler Angles to  Direction Cosine Matrix2/A23 ==
  sin_cos : Inport
  Demux : Demux  Outputs=6
  Terminator{,1..3} (4 alike) : Terminator
  u(1)*u(3) : Product  RndMeth=Zero
  A23 : Outport
  wires:
  Demux/4 -> Terminator/1
  Demux/3 -> Terminator2/1
  Demux/5 -> u(1)*u(3)/2
  Demux/2 -> Terminator3/1
  Demux/1 -> u(1)*u(3)/1
  sin_cos/1 -> Demux/1
  u(1)*u(3)/1 -> A23/1
  Demux/6 -> Terminator1/1

== system controlMCUSlugsMKII/get Nav Vars/Euler Angles to  Direction Cosine Matrix2/A31 ==
  sin_cos : Inport
  Demux : Demux  Outputs=6
  Sum : Sum  Inputs=|++
  Terminator : Terminator
  u(1)*u(3) : Product  RndMeth=Zero
  u(2)*u(4)*u(6) : Product  Inputs=3  RndMeth=Zero
  A31 : Outport
  wires:
  u(1)*u(3)/1 -> Sum/1
  Demux/6 -> u(2)*u(4)*u(6)/3
  Sum/1 -> A31/1
  u(2)*u(4)*u(6)/1 -> Sum/2
  sin_cos/1 -> Demux/1
  Demux/1 -> u(1)*u(3)/1
  Demux/2 -> u(2)*u(4)*u(6)/1
  Demux/5 -> Terminator/1
  Demux/3 -> u(1)*u(3)/2
  Demux/4 -> u(2)*u(4)*u(6)/2

== system controlMCUSlugsMKII/get Nav Vars/Euler Angles to  Direction Cosine Matrix2/A32 ==
  sin_cos : Inport
  Demux : Demux  Outputs=6
  Sum : Sum  Inputs=|+-
  Terminator : Terminator
  u(1)*u(6) : Product  RndMeth=Zero
  u(2)*u(3)*u(4) : Product  Inputs=3  RndMeth=Zero
  A32 : Outport
  wires:
  Demux/4 -> u(2)*u(3)*u(4)/3
  Demux/3 -> u(2)*u(3)*u(4)/2
  Demux/5 -> Terminator/1
  Demux/2 -> u(2)*u(3)*u(4)/1
  Demux/1 -> u(1)*u(6)/2
  sin_cos/1 -> Demux/1
  u(2)*u(3)*u(4)/1 -> Sum/1
  u(1)*u(6)/1 -> Sum/2
  Sum/1 -> A32/1
  Demux/6 -> u(1)*u(6)/1

== system controlMCUSlugsMKII/get Nav Vars/Euler Angles to  Direction Cosine Matrix2/A33 ==
  sin_cos : Inport
  Demux : Demux  Outputs=6
  Terminator{,1..3} (4 alike) : Terminator
  u(4)*u(5) : Product  RndMeth=Zero
  A33 : Outport
  wires:
  Demux/6 -> Terminator/1
  u(4)*u(5)/1 -> A33/1
  sin_cos/1 -> Demux/1
  Demux/1 -> Terminator2/1
  Demux/2 -> Terminator3/1
  Demux/5 -> u(4)*u(5)/2
  Demux/3 -> Terminator1/1
  Demux/4 -> u(4)*u(5)/1

== system controlMCUSlugsMKII/get Nav Vars/Euler Angles to  Direction Cosine Matrix2/Create Transformation Matrix ==
  M11 : Inport
  M12 : Inport  Port=2
  M13 : Inport  Port=3
  M21 : Inport  Port=4
  M22 : Inport  Port=5
  M23 : Inport  Port=6
  M31 : Inport  Port=7
  M32 : Inport  Port=8
  M33 : Inport  Port=9
  Reshape (9) to [3x3] column-major : Reshape  OutputDimensionality=Customize  OutputDimensions=[3,3]
  myMux Fun1 : Stateflow chart
  Matrix : Outport
  wires:
  M33/1 -> myMux Fun1/9(u9)
  M23/1 -> myMux Fun1/8(u8)
  M13/1 -> myMux Fun1/7(u7)
  M32/1 -> myMux Fun1/6(u6)
  Reshape (9) to [3x3] column-major/1 -> Matrix/1
  M22/1 -> myMux Fun1/5(u5)
  M12/1 -> myMux Fun1/4(u4)
  M31/1 -> myMux Fun1/3(u3)
  M21/1 -> myMux Fun1/2(u2)
  M11/1 -> myMux Fun1/1(u1)
  myMux Fun1/1(y) -> Reshape (9) to [3x3] column-major/1

== system controlMCUSlugsMKII/get Nav Vars/Euler Angles to  Direction Cosine Matrix2/Subsystem5 ==
  u : Inport
  C Function Call : dsPICdrivers/OTHERS/C Function Call  Tag=dsPIC_dsPIC_CFunctionCall  fctName='mySin'  INPUT_SIZE=1  INPUT1=real32  INPUT2=--  INPUT3=--  OUTPUT_SIZE=1  OUTPUT1=real32  SampleTime=-1  InputType=[ 7 ]  OutputType=[ 7 ]  FctDeclaration=extern real32_T mySin(real32_T u1);  FctCall=%y1 = mySin(%u1);  OrderingInOutPopup=None
  C Function Call1 : dsPICdrivers/OTHERS/C Function Call  Tag=dsPIC_dsPIC_CFunctionCall  fctName='myCos'  INPUT_SIZE=1  INPUT1=real32  INPUT2=--  INPUT3=--  OUTPUT_SIZE=1  OUTPUT1=real32  SampleTime=-1  InputType=[ 7 ]  OutputType=[ 7 ]  FctDeclaration=extern real32_T myCos(real32_T u1);  FctCall=%y1 = myCos(%u1);  OrderingInOutPopup=None
  C Function Call2 : dsPICdrivers/OTHERS/C Function Call  Tag=dsPIC_dsPIC_CFunctionCall  fctName='mySin'  INPUT_SIZE=1  INPUT1=real32  INPUT2=--  INPUT3=--  OUTPUT_SIZE=1  OUTPUT1=real32  SampleTime=-1  InputType=[ 7 ]  OutputType=[ 7 ]  FctDeclaration=extern real32_T mySin(real32_T u1);  FctCall=%y1 = mySin(%u1);  OrderingInOutPopup=None
  C Function Call3 : dsPICdrivers/OTHERS/C Function Call  Tag=dsPIC_dsPIC_CFunctionCall  fctName='mySin'  INPUT_SIZE=1  INPUT1=real32  INPUT2=--  INPUT3=--  OUTPUT_SIZE=1  OUTPUT1=real32  SampleTime=-1  InputType=[ 7 ]  OutputType=[ 7 ]  FctDeclaration=extern real32_T mySin(real32_T u1);  FctCall=%y1 = mySin(%u1);  OrderingInOutPopup=None
  C Function Call4 : dsPICdrivers/OTHERS/C Function Call  Tag=dsPIC_dsPIC_CFunctionCall  fctName='myCos'  INPUT_SIZE=1  INPUT1=real32  INPUT2=--  INPUT3=--  OUTPUT_SIZE=1  OUTPUT1=real32  SampleTime=-1  InputType=[ 7 ]  OutputType=[ 7 ]  FctDeclaration=extern real32_T myCos(real32_T u1);  FctCall=%y1 = myCos(%u1);  OrderingInOutPopup=None
  C Function Call5 : dsPICdrivers/OTHERS/C Function Call  Tag=dsPIC_dsPIC_CFunctionCall  fctName='myCos'  INPUT_SIZE=1  INPUT1=real32  INPUT2=--  INPUT3=--  OUTPUT_SIZE=1  OUTPUT1=real32  SampleTime=-1  InputType=[ 7 ]  OutputType=[ 7 ]  FctDeclaration=extern real32_T myCos(real32_T u1);  FctCall=%y1 = myCos(%u1);  OrderingInOutPopup=None
  Demux : Demux  Outputs=3
  Demux1 : Demux  Outputs=3
  Environment Controller : simulink/Signal Routing/Environment Controller  SystemSampleTime=-1
  Environment Controller1 : simulink/Signal Routing/Environment Controller  SystemSampleTime=-1
  SinCos1 : aerolibutil/SinCos  SystemSampleTime=-1
  myMux Fun1 : Stateflow chart
  myMux Fun2 : Stateflow chart
  sin(u) : Outport
  cos(u) : Outport  Port=2
  wires:
  myMux Fun2/1(y) -> Environment Controller1/2
  myMux Fun1/1(y) -> Environment Controller/2
  Demux1/3 -> C Function Call5/1
  Demux1/2 -> C Function Call4/1
  Demux1/1 -> C Function Call1/1
  Demux/3 -> C Function Call3/1
  Demux/2 -> C Function Call2/1
  Demux/1 -> C Function Call/1
  C Function Call5/1 -> myMux Fun2/3(u3)
  C Function Call4/1 -> myMux Fun2/2(u2)
  C Function Call1/1 -> myMux Fun2/1(u1)
  C Function Call3/1 -> myMux Fun1/3(u3)
  C Function Call2/1 -> myMux Fun1/2(u2)
  C Function Call/1 -> myMux Fun1/1(u1)
  SinCos1/2 -> Environment Controller1/1
  Environment Controller1/1 -> cos(u)/1
  u/1 -> Demux1/1, Demux/1, SinCos1/1
  SinCos1/1 -> Environment Controller/1
  Environment Controller/1 -> sin(u)/1

== system controlMCUSlugsMKII/Inner Loop/ Navigation/L1 Output Feedback Controller With  Projection Operator/Control  Law/Compute Coef ==
  a : Inport
  Enable : EnablePort
  -T : Gain  Gain=-apSampleTime  SampleTime=apSampleTime
  1-c : Sum  Inputs=-+  OutDataTypeMode=single  OutScaling=2^-10  SampleTime=apSampleTime
  Constant : Constant
  Subsystem11 : Subsystem  AncestorBlock=SLUGS_Library/Subsystem11
  b : Outport
  c : Outport  Port=2
  wires:
  -T/1 -> Subsystem11/1(u)
  Subsystem11/1(exp(u)) -> 1-c/1, c/1  "c"
  Constant/1 -> 1-c/2
  1-c/1 -> b/1
  a/1 -> -T/1

== system controlMCUSlugsMKII/Inner Loop/ Navigation/L1 Output Feedback Controller With  Projection Operator/Control  Law/Detect Change ==
  Data : Inport
  Abs1 : Abs  SampleTime=apSampleTime
  Difference1 : simulink/Discrete/Difference  SystemSampleTime=-1  ICPrevInput=0.0  OutDataType=sfix(16)  OutScaling=2^-10  DoSatur=off
  Saturation1 : Saturate  UpperLimit=1  LowerLimit=0  SampleTime=apSampleTime
  change? : Outport
  wires:
  Difference1/1 -> Abs1/1
  Abs1/1 -> Saturation1/1
  Data/1 -> Difference1/1
  Saturation1/1 -> change?/1

== system controlMCUSlugsMKII/Inner Loop/ Navigation/L1 Output Feedback Controller With  Projection Operator/Projection Operator/Enabled Subsystem ==
  In1 : Inport
  Enable : EnablePort
  Out1 : Outport
  wires:
  In1/1 -> Out1/1

== system controlMCUSlugsMKII/Inner Loop/ Navigation/L1 Output Feedback Controller With  Projection Operator/Projection Operator/Enabled Subsystem1 ==
  y : Inport
  f_the : Inport  Port=2
  grad : Inport  Port=3
  Enable : EnablePort
  Constant : Constant  OutDataTypeMode=single
  Divide1 : Product  OutDataTypeMode=single  OutScaling=2^-10
  Divide2 : Product  OutDataTypeMode=single  OutScaling=2^-10
  Sign : Signum
  Subtract : Sum  Inputs=+-  OutDataTypeMode=single  OutScaling=2^-10
  Out1 : Outport
  wires:
  Divide1/1 -> Subtract/2
  grad/1 -> Sign/1
  Sign/1 -> Divide1/2
  Constant/1 -> Subtract/1
  f_the/1 -> Divide1/1
  Subtract/1 -> Divide2/2
  y/1 -> Divide2/1
  Divide2/1 -> Out1/1

== system controlMCUSlugsMKII/Inner Loop/ Navigation/L1 Output Feedback Controller With  Projection Operator/Projection Operator/F(theta) ==
  Theta Max : Inport
  Eps 0 : Inport  Port=2
  Theta : Inport  Port=3
  Constant : Constant  Value=2  OutDataTypeMode=single
  Divide : Product  OutDataTypeMode=single  OutScaling=2^-10
  Divide1 : Product  OutDataTypeMode=single  OutScaling=2^-10
  Divide2 : Product  OutDataTypeMode=single  OutScaling=2^-10
  Divide3 : Product  Inputs=*/  OutDataTypeMode=single  OutScaling=2^-10
  Divide4 : Product  Inputs=/**  OutDataTypeMode=single  OutScaling=2^-10
  Subtract : Sum  Inputs=+-  OutDataTypeMode=single  OutScaling=2^-10
  "Theta " : InportShadow  Port=3  LatchByCopyingInsideSignal=off
  f_theta : Outport
  dif_f_theta : Outport  Port=2
  wires:
  Theta/1 -> Divide/1, Divide/2
  Theta Max/1 -> Divide1/2, Divide1/1
  Divide/1 -> Subtract/1
  Divide1/1 -> Subtract/2, Divide2/1
  Eps 0/1 -> Divide2/2
  Subtract/1 -> Divide3/1
  Divide2/1 -> Divide3/2, Divide4/1
  Divide3/1 -> f_theta/1
  Constant/1 -> Divide4/3
  "Theta "/1 -> Divide4/2
  Divide4/1 -> dif_f_theta/1

== system controlMCUSlugsMKII/Inner Loop/ Navigation/L1 Output Feedback Controller With  Projection Operator/State Predictor/Compute Coef ==
  a : Inport
  Enable : EnablePort
  -T : Gain  Gain=-apSampleTime  SampleTime=apSampleTime
  1-c : Sum  Inputs=-+  OutDataTypeMode=single  OutScaling=2^-10
  Constant : Constant
  Subsystem11 : Subsystem  AncestorBlock=SLUGS_Library/Subsystem11
  b : Outport
  c : Outport  Port=2
  wires:
  a/1 -> -T/1
  1-c/1 -> b/1
  Constant/1 -> 1-c/2
  Subsystem11/1(exp(u)) -> c/1, 1-c/1  "c"
  -T/1 -> Subsystem11/1(u)

== system controlMCUSlugsMKII/Inner Loop/ Navigation/L1 Output Feedback Controller With  Projection Operator/State Predictor/Detect Change ==
  Data : Inport
  Abs1 : Abs  SampleTime=apSampleTime
  Difference1 : simulink/Discrete/Difference  SystemSampleTime=-1  ICPrevInput=0.0  OutDataType=sfix(16)  OutScaling=2^-10  DoSatur=off
  Saturation1 : Saturate  UpperLimit=1  LowerLimit=0  SampleTime=apSampleTime
  change? : Outport
  wires:
  Saturation1/1 -> change?/1
  Data/1 -> Difference1/1
  Abs1/1 -> Saturation1/1
  Difference1/1 -> Abs1/1

== system controlMCUSlugsMKII/Inner Loop/ Navigation/L1 Output Feedback Controller With  Projection Operator/Trapezoidal Integrator/Protect NaNs ==
  In1 : Inport
  Integer Delay3 : simulink/Discrete/Integer Delay  Orientation=left  vinit=0.0  samptime=T  NumDelays=1
  Relational Operator2 : RelationalOperator  Operator===  LogicOutDataTypeMode=Specify via dialog
  Switch3 : Switch  Criteria=u2 > Threshold  Threshold=0.3  SampleTime=.01
  Out1 : Outport  Orientation=down
  wires:
  Relational Operator2/1 -> Switch3/2
  In1/1 -> Switch3/1, Relational Operator2/1, Relational Operator2/2
  Switch3/1 -> Integer Delay3/1, Out1/1
  Integer Delay3/1 -> Switch3/3

== system controlMCUSlugsMKII/Inner Loop/ Navigation/L1 Output Feedback Controller With  Projection Operator/Trapezoidal Integrator/Protect NaNs1 ==
  In1 : Inport
  Integer Delay3 : simulink/Discrete/Integer Delay  Orientation=left  vinit=0.0  samptime=T  NumDelays=1
  Relational Operator2 : RelationalOperator  Operator===  LogicOutDataTypeMode=Specify via dialog
  Switch3 : Switch  Criteria=u2 > Threshold  Threshold=0.3  SampleTime=.01
  Out1 : Outport  Orientation=down
  wires:
  Integer Delay3/1 -> Switch3/3
  Switch3/1 -> Out1/1, Integer Delay3/1
  In1/1 -> Relational Operator2/2, Relational Operator2/1, Switch3/1
  Relational Operator2/1 -> Switch3/2

== system controlMCUSlugsMKII/Inner Loop/ Navigation/Lateral Channel/Bank to Psi Dot/Protect NaNs ==
  In1 : Inport
  Integer Delay3 : simulink/Discrete/Integer Delay  Orientation=left  vinit=0.0  samptime=T  NumDelays=1
  Relational Operator2 : RelationalOperator  Operator===  LogicOutDataTypeMode=Specify via dialog
  Switch3 : Switch  Criteria=u2 > Threshold  Threshold=0.3  SampleTime=.01
  Out1 : Outport  Orientation=down
  wires:
  Relational Operator2/1 -> Switch3/2
  In1/1 -> Switch3/1, Relational Operator2/1, Relational Operator2/2
  Switch3/1 -> Integer Delay3/1, Out1/1
  Integer Delay3/1 -> Switch3/3
